simulink model "exampleHelperAvoidObstaclesMobileRobot"  (R2023b)
settings: Solver=VariableStepAuto  StartTime=0.0  StopTime=inf  RelTol=1e-3
undefined symbols (not defined in the file or in its folder): initTheta, initX, initY, lidarNoiseSeeds, lidarNoiseVariance, mapMatrix, maxAngSpeed, maxLinSpeed, maxRange, sampleTime
libraries: simulink x3, rllib x1, robotmobilelib x1
settings Model: Creator=The MathWorks, Inc.  LastModifiedBy=pc
settings SolverCC: AlgebraicLoopSolver=TrustRegion
settings DebuggingCC: UnconnectedInputMsg=warning  UnconnectedOutputMsg=warning  UnconnectedLineMsg=warning
settings ModelReferenceCC: EnableRefExpFcnMdlSchedulingChecks=on

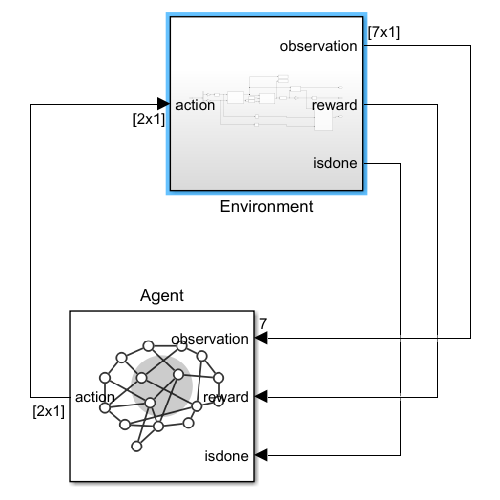
[thumbnail: Simulink's stored preview of the top-level diagram]
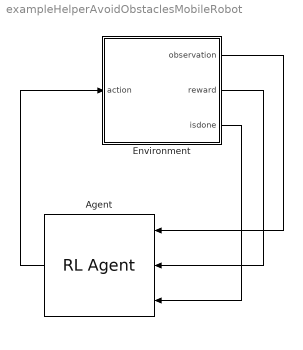
== system exampleHelperAvoidObstaclesMobileRobot ==
  Agent : rllib/RL Agent  Agent=obstacleAvoidanceAgent  ExternalActionAsInput=off  ProvideLastAction=off  ProvideCumRwd=off  TreatAsDirectFeedthrough=on  UseStrictObservationDataTypes=off
  Environment : Subsystem
  wires:
  Environment/1(observation) -> Agent/1
  Environment/2(reward) -> Agent/2
  Environment/3(isdone) -> Agent/3
  Agent/1 -> Environment/1(action)

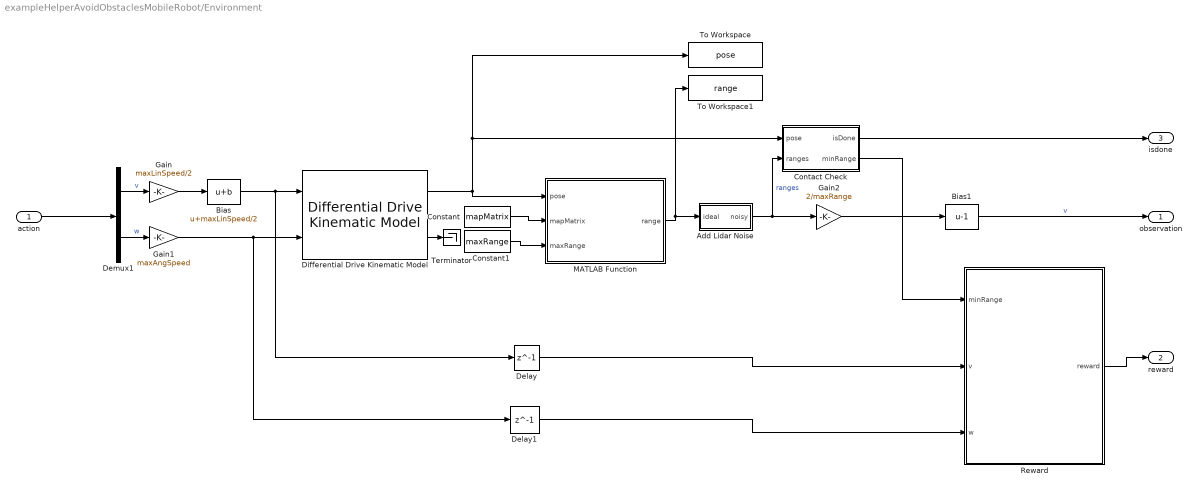
== system exampleHelperAvoidObstaclesMobileRobot/Environment ==
  action : Inport
  Add Lidar Noise : Subsystem
  Bias : Bias  Bias=maxLinSpeed/2  SaturateOnIntegerOverflow=off
  Bias1 : Bias  Bias=-1  SaturateOnIntegerOverflow=off
  Constant : Constant  Value=mapMatrix
  Constant1 : Constant  Value=maxRange
  Contact Check : Subsystem
  Delay : Delay  DelayLength=1  InitialCondition=0  UseCircularBuffer=on
  Delay1 : Delay  DelayLength=1  InitialCondition=0  UseCircularBuffer=on
  Demux1 : Demux  Outputs=2
  Differential Drive Kinematic Model : robotmobilelib/Differential Drive Kinematic Model  VehicleInputs=Vehicle Speed & Heading Angular Velocity  WheelRadius=0.05  WheelSpeedRange=[-inf inf]  TrackWidth=0.2  InitialState=[initX; initY; initTheta]  SimulateUsing=Code generation
  Gain : Gain  Gain=maxLinSpeed/2
  Gain1 : Gain  Gain=maxAngSpeed
  Gain2 : Gain  Gain=2/maxRange
  MATLAB Function : MATLAB Function  TreatAsAtomicUnit=on
  Reward : Subsystem
  Terminator : Terminator
  To Workspace : ToWorkspace  VariableName=pose  SampleTime=-1
      settings: Save2DSignal=2-D array (concatenate along first dimension)
  To Workspace1 : ToWorkspace  VariableName=range  SampleTime=-1
  observation : Outport
  reward : Outport  Port=2
  isdone : Outport  Port=3
  wires:
  Differential Drive Kinematic Model/2 -> Terminator/1
  Constant/1 -> MATLAB Function/2(mapMatrix)
  Differential Drive Kinematic Model/1 -> To Workspace/1, Contact Check/1(pose), MATLAB Function/1(pose)
  action/1 -> Demux1/1
  Bias/1 -> Delay/1, Differential Drive Kinematic Model/1
  Gain1/1 -> Delay1/1, Differential Drive Kinematic Model/2
  MATLAB Function/1(range) -> To Workspace1/1, Add Lidar Noise/1(ideal)
  Contact Check/1(isDone) -> isdone/1
  Contact Check/2(minRange) -> Reward/1(minRange)
  Reward/1(reward) -> reward/1
  Gain2/1 -> Bias1/1
  Bias1/1 -> observation/1  "v"
  Constant1/1 -> MATLAB Function/3(maxRange)
  Delay/1 -> Reward/2(v)
  Delay1/1 -> Reward/3(w)
  Demux1/2 -> Gain1/1  "w"
  Gain/1 -> Bias/1
  Demux1/1 -> Gain/1  "v"
  Add Lidar Noise/1(noisy) -> Gain2/1, Contact Check/2(ranges)  "ranges"

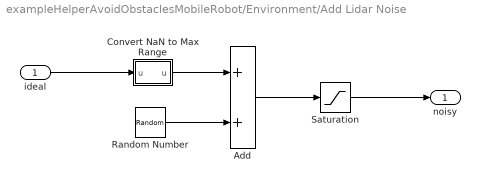
== system exampleHelperAvoidObstaclesMobileRobot/Environment/Add Lidar Noise ==
  ideal : Inport
  Add : Sum
  Convert NaN to Max Range : MATLAB Function  TreatAsAtomicUnit=on
  Random Number : RandomNumber  Variance=lidarNoiseVariance  Seed=lidarNoiseSeeds  SampleTime=sampleTime
  Saturation : Saturate  UpperLimit=inf  LowerLimit=0
  noisy : Outport
  wires:
  Random Number/1 -> Add/2
  Add/1 -> Saturation/1
  Saturation/1 -> noisy/1
  ideal/1 -> Convert NaN to Max Range/1("u ")
  Convert NaN to Max Range/1(u) -> Add/1

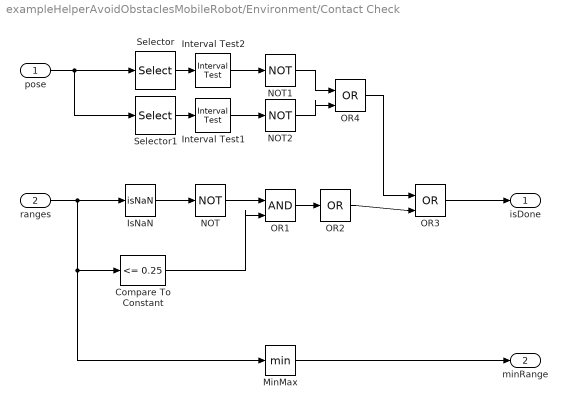
== system exampleHelperAvoidObstaclesMobileRobot/Environment/Contact Check ==
  pose : Inport
  ranges : Inport  Port=2
  Compare To Constant : simulink/Logic and Bit Operations/Compare To Constant  relop=<=  const=0.25  OutDataTypeStr=boolean
  Interval Test1 : simulink/Logic and Bit Operations/Interval Test  IntervalClosedRight=on  uplimit=size(mapMatrix, 1)  IntervalClosedLeft=on  lowlimit=0  OutDataTypeStr=boolean
  Interval Test2 : simulink/Logic and Bit Operations/Interval Test  IntervalClosedRight=on  uplimit=size(mapMatrix, 2)  IntervalClosedLeft=on  lowlimit=0  OutDataTypeStr=boolean
  IsNaN : RelationalOperator  Operator=isNaN  OutDataTypeStr=boolean  RndMeth=Simplest  InputSameDT=off
  MinMax : MinMax
  NOT : Logic  Operator=NOT  IconShape=distinctive  AllPortsSameDT=off  OutDataTypeStr=boolean
  NOT1 : Logic  Operator=NOT  IconShape=distinctive  AllPortsSameDT=off  OutDataTypeStr=boolean
  NOT2 : Logic  Operator=NOT  IconShape=distinctive  AllPortsSameDT=off  OutDataTypeStr=boolean
  OR1 : Logic  IconShape=distinctive  AllPortsSameDT=off  OutDataTypeStr=boolean
  OR2 : Logic  Operator=OR  Inputs=1  IconShape=distinctive  AllPortsSameDT=off  OutDataTypeStr=boolean
  OR3 : Logic  Operator=OR  IconShape=distinctive  AllPortsSameDT=off  OutDataTypeStr=boolean
  OR4 : Logic  Operator=OR  IconShape=distinctive  AllPortsSameDT=off  OutDataTypeStr=boolean
  Selector : Selector  InputPortWidth=3  IndexOptions=Index vector (dialog)  Indices=1  OutputSizes=1
  Selector1 : Selector  InputPortWidth=3  IndexOptions=Index vector (dialog)  Indices=2  OutputSizes=1
  isDone : Outport  VectorParamsAs1DForOutWhenUnconnected=off
  minRange : Outport  Port=2  VectorParamsAs1DForOutWhenUnconnected=off
  wires:
  OR1/1 -> OR2/1
  Compare To Constant/1 -> OR1/2
  NOT/1 -> OR1/1
  ranges/1 -> MinMax/1, Compare To Constant/1, IsNaN/1
  IsNaN/1 -> NOT/1
  MinMax/1 -> minRange/1
  OR3/1 -> isDone/1
  pose/1 -> Selector/1, Selector1/1
  Selector/1 -> Interval Test2/1
  Selector1/1 -> Interval Test1/1
  OR2/1 -> OR3/2
  NOT1/1 -> OR4/1
  Interval Test1/1 -> NOT2/1
  OR4/1 -> OR3/1
  Interval Test2/1 -> NOT1/1
  NOT2/1 -> OR4/2

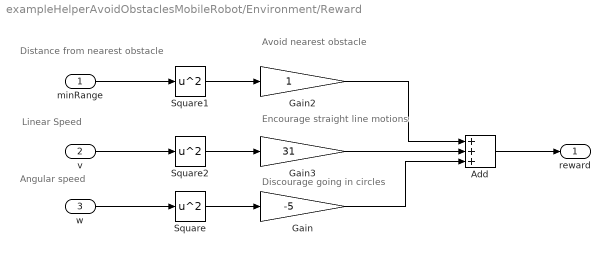
== system exampleHelperAvoidObstaclesMobileRobot/Environment/Reward ==
  note: Discourage going in circles
  note: Encourage straight line motions
  note: Angular speed
  note: Linear Speed
  note: Distance from nearest obstacle
  note: Avoid nearest obstacle
  minRange : Inport
  v : Inport  Port=2
  w : Inport  Port=3
  Add : Sum  Inputs=+++
  Gain : Gain  Gain=-5
  Gain2 : Gain
  Gain3 : Gain  Gain=31
  Square : Math  Operator=square  SignedPower=on
  Square1 : Math  Operator=square  SignedPower=on
  Square2 : Math  Operator=square  SignedPower=on
  reward : Outport  VectorParamsAs1DForOutWhenUnconnected=off
  wires:
  Square/1 -> Gain/1
  w/1 -> Square/1
  Gain/1 -> Add/3
  minRange/1 -> Square1/1
  Gain2/1 -> Add/1
  Square1/1 -> Gain2/1
  v/1 -> Square2/1
  Square2/1 -> Gain3/1
  Gain3/1 -> Add/2
  Add/1 -> reward/1

== matlab function exampleHelperAvoidObstaclesMobileRobot/Environment/MATLAB Function ==
  settings: updateMethod=DISCRETE
  data: range output size=[7, 1]; pose input size=[3, 1]; mapMatrix input size=[size(mapMatrix, 1), size(mapMatrix, 2)]; maxRange input; mapScale parameter
function range = RangeSensor(pose, mapMatrix, maxRange, mapScale)
range=exampleHelperAvoidObstaclesRangeSensor(pose,mapMatrix,maxRange,mapScale);

== matlab function exampleHelperAvoidObstaclesMobileRobot/Environment/Add Lidar Noise/Convert NaN to Max Range ==
  data: u input; u output; maxRange parameter
function u = removeNans(u,maxRange)

u(isnan(u)) = maxRange;
